simulink model "REGISTROS_64_BITS_01"  (R2022a)
settings: Solver=VariableStepAuto  StartTime=0.0  StopTime=10.0  RelTol=1e-3
undefined symbols (not defined in the file or in its folder): xc7z010iclg225
libraries: hdlBasic x6608, vmcUtilities x1
(part 1 of 23)
settings Model: Creator=sebas  LastModifiedBy=sebas

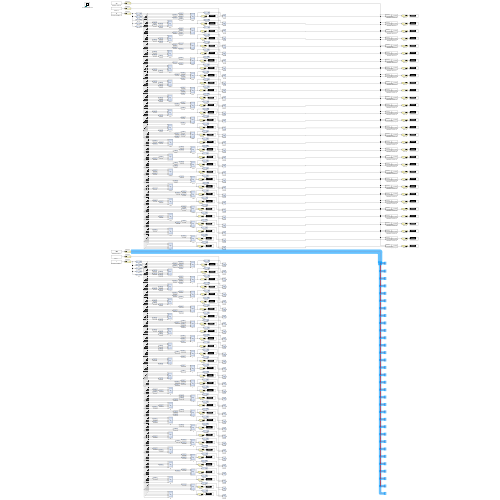
[thumbnail: Simulink's stored preview of the top-level diagram]
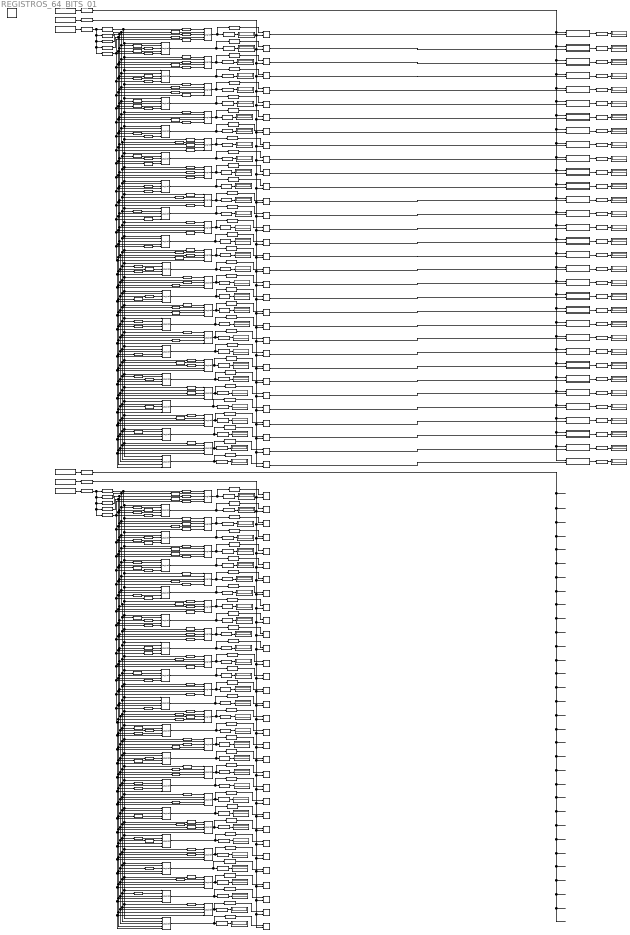
== system REGISTROS_64_BITS_01 ==
  00000 : hdlBasic/Logical  logical_function=AND  inputs=5  en=off  latency=0  precision=Full  arith_type=Unsigned  n_bits=16  bin_pt=0  align_bp=on  overflow=[]  quantization=[]  XmcBlockStatus=1  maskContainerNames=tabcontainer1  block_type=logical  block_config=sysgen:Logical_config
  00001 : hdlBasic/Logical  logical_function=AND  inputs=5  en=off  latency=0  precision=Full  arith_type=Unsigned  n_bits=16  bin_pt=0  align_bp=on  overflow=[]  quantization=[]  XmcBlockStatus=1  maskContainerNames=tabcontainer1  block_type=logical  block_config=sysgen:Logical_config
  00010 : hdlBasic/Logical  logical_function=AND  inputs=5  en=off  latency=0  precision=Full  arith_type=Unsigned  n_bits=16  bin_pt=0  align_bp=on  overflow=[]  quantization=[]  XmcBlockStatus=1  maskContainerNames=tabcontainer1  block_type=logical  block_config=sysgen:Logical_config
  00011 : hdlBasic/Logical  logical_function=AND  inputs=5  en=off  latency=0  precision=Full  arith_type=Unsigned  n_bits=16  bin_pt=0  align_bp=on  overflow=[]  quantization=[]  XmcBlockStatus=1  maskContainerNames=tabcontainer1  block_type=logical  block_config=sysgen:Logical_config
  00100 : hdlBasic/Logical  logical_function=AND  inputs=5  en=off  latency=0  precision=Full  arith_type=Unsigned  n_bits=16  bin_pt=0  align_bp=on  overflow=[]  quantization=[]  XmcBlockStatus=1  maskContainerNames=tabcontainer1  block_type=logical  block_config=sysgen:Logical_config
  00101 : hdlBasic/Logical  logical_function=AND  inputs=5  en=off  latency=0  precision=Full  arith_type=Unsigned  n_bits=16  bin_pt=0  align_bp=on  overflow=[]  quantization=[]  XmcBlockStatus=1  maskContainerNames=tabcontainer1  block_type=logical  block_config=sysgen:Logical_config
  00110 : hdlBasic/Logical  logical_function=AND  inputs=5  en=off  latency=0  precision=Full  arith_type=Unsigned  n_bits=16  bin_pt=0  align_bp=on  overflow=[]  quantization=[]  XmcBlockStatus=1  maskContainerNames=tabcontainer1  block_type=logical  block_config=sysgen:Logical_config
  00111 : hdlBasic/Logical  logical_function=AND  inputs=5  en=off  latency=0  precision=Full  arith_type=Unsigned  n_bits=16  bin_pt=0  align_bp=on  overflow=[]  quantization=[]  XmcBlockStatus=1  maskContainerNames=tabcontainer1  block_type=logical  block_config=sysgen:Logical_config
  01000 : hdlBasic/Logical  logical_function=AND  inputs=5  en=off  latency=0  precision=Full  arith_type=Unsigned  n_bits=16  bin_pt=0  align_bp=on  overflow=[]  quantization=[]  XmcBlockStatus=1  maskContainerNames=tabcontainer1  block_type=logical  block_config=sysgen:Logical_config
  01001 : hdlBasic/Logical  logical_function=AND  inputs=5  en=off  latency=0  precision=Full  arith_type=Unsigned  n_bits=16  bin_pt=0  align_bp=on  overflow=[]  quantization=[]  XmcBlockStatus=1  maskContainerNames=tabcontainer1  block_type=logical  block_config=sysgen:Logical_config
  01010 : hdlBasic/Logical  logical_function=AND  inputs=5  en=off  latency=0  precision=Full  arith_type=Unsigned  n_bits=16  bin_pt=0  align_bp=on  overflow=[]  quantization=[]  XmcBlockStatus=1  maskContainerNames=tabcontainer1  block_type=logical  block_config=sysgen:Logical_config
  01011 : hdlBasic/Logical  logical_function=AND  inputs=5  en=off  latency=0  precision=Full  arith_type=Unsigned  n_bits=16  bin_pt=0  align_bp=on  overflow=[]  quantization=[]  XmcBlockStatus=1  maskContainerNames=tabcontainer1  block_type=logical  block_config=sysgen:Logical_config
  01100 : hdlBasic/Logical  logical_function=AND  inputs=5  en=off  latency=0  precision=Full  arith_type=Unsigned  n_bits=16  bin_pt=0  align_bp=on  overflow=[]  quantization=[]  XmcBlockStatus=1  maskContainerNames=tabcontainer1  block_type=logical  block_config=sysgen:Logical_config
  01101 : hdlBasic/Logical  logical_function=AND  inputs=5  en=off  latency=0  precision=Full  arith_type=Unsigned  n_bits=16  bin_pt=0  align_bp=on  overflow=[]  quantization=[]  XmcBlockStatus=1  maskContainerNames=tabcontainer1  block_type=logical  block_config=sysgen:Logical_config
  01110 : hdlBasic/Logical  logical_function=AND  inputs=5  en=off  latency=0  precision=Full  arith_type=Unsigned  n_bits=16  bin_pt=0  align_bp=on  overflow=[]  quantization=[]  XmcBlockStatus=1  maskContainerNames=tabcontainer1  block_type=logical  block_config=sysgen:Logical_config
  01111 : hdlBasic/Logical  logical_function=AND  inputs=5  en=off  latency=0  precision=Full  arith_type=Unsigned  n_bits=16  bin_pt=0  align_bp=on  overflow=[]  quantization=[]  XmcBlockStatus=1  maskContainerNames=tabcontainer1  block_type=logical  block_config=sysgen:Logical_config
  {1..32,10000..10001,10010..10011,10100..10101,10110..10111,11000..11001,11010..11011,11100..11101,11110..11111} (48 alike) : hdlBasic/Logical  logical_function=AND  inputs=5  en=off  latency=0  precision=Full  arith_type=Unsigned  n_bits=16  bin_pt=0  align_bp=on  overflow=[]  quantization=[]  XmcBlockStatus=1  maskContainerNames=tabcontainer1  block_type=logical  block_config=sysgen:Logical_config
  BIT_00 : hdlBasic/Slice  nbits=1  boolean_output=off  mode=Lower Bit Location + Width  bit1=-3  base1=MSB of Input  bit0=0  base0=LSB of Input  XmcBlockStatus=1  maskContainerNames=group1  block_type=slice  block_config=sysgen:Slice_config
  BIT_01 : hdlBasic/Slice  nbits=1  boolean_output=off  mode=Lower Bit Location + Width  bit1=-2  base1=MSB of Input  bit0=1  base0=LSB of Input  XmcBlockStatus=1  maskContainerNames=group1  block_type=slice  block_config=sysgen:Slice_config
  BIT_02 : hdlBasic/Slice  nbits=1  boolean_output=off  mode=Lower Bit Location + Width  bit1=-3  base1=MSB of Input  bit0=2  base0=LSB of Input  XmcBlockStatus=1  maskContainerNames=group1  block_type=slice  block_config=sysgen:Slice_config
  BIT_03 : hdlBasic/Slice  nbits=1  boolean_output=off  mode=Lower Bit Location + Width  bit1=-2  base1=MSB of Input  bit0=3  base0=LSB of Input  XmcBlockStatus=1  maskContainerNames=group1  block_type=slice  block_config=sysgen:Slice_config
  BIT_04 : hdlBasic/Slice  nbits=1  boolean_output=off  mode=Lower Bit Location + Width  bit1=-2  base1=MSB of Input  bit0=4  base0=LSB of Input  XmcBlockStatus=1  maskContainerNames=group1  block_type=slice  block_config=sysgen:Slice_config
  BIT_1 : hdlBasic/Slice  nbits=1  boolean_output=off  mode=Lower Bit Location + Width  bit1=-3  base1=MSB of Input  bit0=0  base0=LSB of Input  XmcBlockStatus=1  maskContainerNames=group1  block_type=slice  block_config=sysgen:Slice_config
  BIT_2 : hdlBasic/Slice  nbits=1  boolean_output=off  mode=Lower Bit Location + Width  bit1=-2  base1=MSB of Input  bit0=1  base0=LSB of Input  XmcBlockStatus=1  maskContainerNames=group1  block_type=slice  block_config=sysgen:Slice_config
  BIT_3 : hdlBasic/Slice  nbits=1  boolean_output=off  mode=Lower Bit Location + Width  bit1=-3  base1=MSB of Input  bit0=2  base0=LSB of Input  XmcBlockStatus=1  maskContainerNames=group1  block_type=slice  block_config=sysgen:Slice_config
  BIT_4 : hdlBasic/Slice  nbits=1  boolean_output=off  mode=Lower Bit Location + Width  bit1=-2  base1=MSB of Input  bit0=3  base0=LSB of Input  XmcBlockStatus=1  maskContainerNames=group1  block_type=slice  block_config=sysgen:Slice_config
  BIT_5 : hdlBasic/Slice  nbits=1  boolean_output=off  mode=Lower Bit Location + Width  bit1=-2  base1=MSB of Input  bit0=4  base0=LSB of Input  XmcBlockStatus=1  maskContainerNames=group1  block_type=slice  block_config=sysgen:Slice_config
  Convert{,1..63} (64 alike) : hdlBasic/Convert  gui_display_data_type=Boolean  arith_type=Boolean  n_bits=16  bin_pt=14  float_type=Single  exp_bits=8  fraction_bits=24  quantization=Truncate  overflow=Wrap  en=off  latency=0  pipeline=off  XmcBlockStatus=1  maskContainerNames=group2  block_type=convert  block_config=sysgen:Convert_config  block_width=595  block_height=885
  Display{1..96} (96 alike) : Display
      Display38 settings: Format=decimal (Stored Integer)
      Display39 settings: Format=decimal (Stored Integer)
      Display40 settings: Format=decimal (Stored Integer)
      Display41 settings: Format=decimal (Stored Integer)
      Display42 settings: Format=decimal (Stored Integer)
      Display43 settings: Format=decimal (Stored Integer)
      Display44 settings: Format=decimal (Stored Integer)
      Display45 settings: Format=decimal (Stored Integer)
      Display46 settings: Format=decimal (Stored Integer)
      Display47 settings: Format=decimal (Stored Integer)
      Display48 settings: Format=decimal (Stored Integer)
      Display49 settings: Format=decimal (Stored Integer)
      Display50 settings: Format=decimal (Stored Integer)
      Display51 settings: Format=decimal (Stored Integer)
      Display52 settings: Format=decimal (Stored Integer)
      Display53 settings: Format=decimal (Stored Integer)
      Display54 settings: Format=decimal (Stored Integer)
      Display55 settings: Format=decimal (Stored Integer)
      Display56 settings: Format=decimal (Stored Integer)
      Display57 settings: Format=decimal (Stored Integer)
      Display58 settings: Format=decimal (Stored Integer)
      Display59 settings: Format=decimal (Stored Integer)
      Display60 settings: Format=decimal (Stored Integer)
      Display61 settings: Format=decimal (Stored Integer)
      Display62 settings: Format=decimal (Stored Integer)
      Display63 settings: Format=decimal (Stored Integer)
      Display64 settings: Format=decimal (Stored Integer)
      Display65 settings: Format=decimal (Stored Integer)
      Display66 settings: Format=decimal (Stored Integer)
      Display67 settings: Format=decimal (Stored Integer)
      Display68 settings: Format=decimal (Stored Integer)
      Display88 settings: Format=decimal (Stored Integer)
  Gateway In1 : hdlBasic/Gateway In  gui_display_data_type=Boolean  arith_type=Boolean  n_bits=1  bin_pt=0  preci_type=Single  exp_width=8  frac_width=24  rows=1  columns=1  quantization="Round  (unbiased: +/- Inf)"  overflow=Saturate  period=1  UseAsADC=off  ADCChannel='1'  interface=None  automatic_assignment=on  address_offset=hex2dec('00')  intf_name=''  intf_description=''  default_value=0  timing_constraint=None  locs_specified=off  LOCs={}  io_standard={}  inherit_from_input=off  hdl_port=on  XmcBlockStatus=1  maskContainerNames=group4  block_type=gatewayin  block_config=sysgen:gateway_in_config  block_width_w=590  block_height_w=620  block_width=640  block_height=850
  Gateway In2 : hdlBasic/Gateway In  gui_display_data_type=Fixed-point  arith_type=Signed (2's comp)  n_bits=64  bin_pt=0  preci_type=Single  exp_width=8  frac_width=24  rows=1  columns=1  quantization="Round  (unbiased: +/- Inf)"  overflow=Saturate  period=1  UseAsADC=off  ADCChannel='1'  interface=None  automatic_assignment=on  address_offset=hex2dec('00')  intf_name=''  intf_description=''  default_value=0  timing_constraint=None  locs_specified=off  LOCs={}  io_standard={}  inherit_from_input=off  hdl_port=on  XmcBlockStatus=1  maskContainerNames=group4  block_type=gatewayin  block_config=sysgen:gateway_in_config  block_width_w=590  block_height_w=620  block_width=640  block_height=850
  Gateway In3 : hdlBasic/Gateway In  gui_display_data_type=Boolean  arith_type=Boolean  n_bits=1  bin_pt=0  preci_type=Single  exp_width=8  frac_width=24  rows=1  columns=1  quantization="Round  (unbiased: +/- Inf)"  overflow=Saturate  period=1  UseAsADC=off  ADCChannel='1'  interface=None  automatic_assignment=on  address_offset=hex2dec('00')  intf_name=''  intf_description=''  default_value=0  timing_constraint=None  locs_specified=off  LOCs={}  io_standard={}  inherit_from_input=off  hdl_port=on  XmcBlockStatus=1  maskContainerNames=group4  block_type=gatewayin  block_config=sysgen:gateway_in_config  block_width_w=590  block_height_w=620  block_width=640  block_height=850
  Gateway In4 : hdlBasic/Gateway In  gui_display_data_type=Fixed-point  arith_type=Signed (2's comp)  n_bits=64  bin_pt=0  preci_type=Single  exp_width=8  frac_width=24  rows=1  columns=1  quantization="Round  (unbiased: +/- Inf)"  overflow=Saturate  period=1  UseAsADC=off  ADCChannel='1'  interface=None  automatic_assignment=on  address_offset=hex2dec('00')  intf_name=''  intf_description=''  default_value=0  timing_constraint=None  locs_specified=off  LOCs={}  io_standard={}  inherit_from_input=off  hdl_port=on  XmcBlockStatus=1  maskContainerNames=group4  block_type=gatewayin  block_config=sysgen:gateway_in_config  block_width_w=590  block_height_w=620  block_width=640  block_height=850
  Gateway In5 : hdlBasic/Gateway In  gui_display_data_type=Fixed-point  arith_type=Unsigned  n_bits=5  bin_pt=0  preci_type=Single  exp_width=8  frac_width=24  rows=1  columns=1  quantization="Round  (unbiased: +/- Inf)"  overflow=Saturate  period=1  UseAsADC=off  ADCChannel='1'  interface=None  automatic_assignment=on  address_offset=hex2dec('00')  intf_name=''  intf_description=''  default_value=0  timing_constraint=None  locs_specified=off  LOCs={}  io_standard={}  inherit_from_input=off  hdl_port=on  XmcBlockStatus=1  maskContainerNames=group4  block_type=gatewayin  block_config=sysgen:gateway_in_config  block_width_w=590  block_height_w=620  block_width=640  block_height=850
  Gateway In9 : hdlBasic/Gateway In  gui_display_data_type=Fixed-point  arith_type=Unsigned  n_bits=5  bin_pt=0  preci_type=Single  exp_width=8  frac_width=24  rows=1  columns=1  quantization="Round  (unbiased: +/- Inf)"  overflow=Saturate  period=1  UseAsADC=off  ADCChannel='1'  interface=None  automatic_assignment=on  address_offset=hex2dec('00')  intf_name=''  intf_description=''  default_value=0  timing_constraint=None  locs_specified=off  LOCs={}  io_standard={}  inherit_from_input=off  hdl_port=on  XmcBlockStatus=1  maskContainerNames=group4  block_type=gatewayin  block_config=sysgen:gateway_in_config  block_width_w=590  block_height_w=620  block_width=640  block_height=850
  Inverter{1..160} (160 alike) : hdlBasic/Inverter  en=off  latency=0  XmcBlockStatus=1  maskContainerNames=group2  block_type=inv  block_config=sysgen:Inverter_config
  Logical{,1..63} (64 alike) : hdlBasic/Logical  logical_function=AND  inputs=2  en=off  latency=0  precision=Full  arith_type=Unsigned  n_bits=16  bin_pt=0  align_bp=on  overflow=[]  quantization=[]  XmcBlockStatus=1  maskContainerNames=tabcontainer1  block_type=logical  block_config=sysgen:Logical_config
  REGISTER_DATA_00 : Constant  Value=99985
  REGISTER_DATA_1 : Constant  Value=99985
  REGISTER_NUMBER_00 : Constant  Value=30
  REGISTER_NUMBER_1 : Constant  Value=30
  REGISTRO_64_BITS_00 : Subsystem
  REGISTRO_64_BITS_1 : Subsystem
  REGISTRO_64_BITS_10 : Subsystem
  REGISTRO_64_BITS_11 : Subsystem
  REGISTRO_64_BITS_12 : Subsystem
  REGISTRO_64_BITS_13 : Subsystem
  REGISTRO_64_BITS_14 : Subsystem
  REGISTRO_64_BITS_15 : Subsystem
  REGISTRO_64_BITS_16 : Subsystem
  REGISTRO_64_BITS_17 : Subsystem
  REGISTRO_64_BITS_18 : Subsystem
  REGISTRO_64_BITS_19 : Subsystem
  REGISTRO_64_BITS_2 : Subsystem
  REGISTRO_64_BITS_20 : Subsystem
  REGISTRO_64_BITS_21 : Subsystem
  REGISTRO_64_BITS_22 : Subsystem
  REGISTRO_64_BITS_23 : Subsystem
  REGISTRO_64_BITS_24 : Subsystem
  REGISTRO_64_BITS_25 : Subsystem
  REGISTRO_64_BITS_26 : Subsystem
  REGISTRO_64_BITS_27 : Subsystem
  REGISTRO_64_BITS_28 : Subsystem
  REGISTRO_64_BITS_29 : Subsystem
  REGISTRO_64_BITS_3 : Subsystem
  REGISTRO_64_BITS_30 : Subsystem
  REGISTRO_64_BITS_31 : Subsystem
  REGISTRO_64_BITS_4 : Subsystem
  REGISTRO_64_BITS_5 : Subsystem
  REGISTRO_64_BITS_6 : Subsystem
  REGISTRO_64_BITS_7 : Subsystem
  REGISTRO_64_BITS_8 : Subsystem
  REGISTRO_64_BITS_9 : Subsystem
  Result{1..64} (64 alike) : hdlBasic/Gateway Out  inherit_from_input=off  hdl_port=on  rows=1  columns=1  UseAsDAC=off  DACChannel='1'  interface=None  automatic_assignment=on  address_offset=hex2dec('00')  intf_name=''  intf_description=''  timing_constraint=None  locs_specified=off  LOCs={}  io_standard={}  XmcBlockStatus=1  maskContainerNames=group4  block_type=gatewayout  block_config=sysgen:gateway_out_config  block_width_w=590  block_height_w=620  block_width=620  block_height=750
  Result_{1..32} (32 alike) : hdlBasic/Gateway Out  inherit_from_input=off  hdl_port=on  rows=1  columns=1  UseAsDAC=off  DACChannel='1'  interface=None  automatic_assignment=on  address_offset=hex2dec('00')  intf_name=''  intf_description=''  timing_constraint=None  locs_specified=off  LOCs={}  io_standard={}  XmcBlockStatus=1  maskContainerNames=group4  block_type=gatewayout  block_config=sysgen:gateway_out_config  block_width_w=590  block_height_w=620  block_width=620  block_height=750
  Vitis Model Composer Hub : vmcUtilities/Vitis Model Composer Hub  Tag=genX  CodeGeneration=off  TargetDirectory=./code  ExportType=AI Engines  IpVendor=xilinx.com  IpLibrary=hls  IpVersion=1.0  IpHWLanguage=Verilog  AieCompilerOptions={}  AieSimulatorOptions={}  CreateTestbench=off  TestbenchStackSize=10  RunAieSim=off  AieSimTimeout=50000  RunAieSimProfiling=off  LaunchVitisAnalyzer=off  PlotOutput=off  RunX86Sim=off  X86SimTimeout=10  GenHwImage=off  PlatformType=Not Specified  HwSystemType=Baremetal  HwValidationTarget=hw  ProjDevice=xc7z010iclg225-1L  ProjDevicePart=xc7z010iclg225-1L  SamplePeriod=-1  ClockFrequency=200  DataPathParallelism=1  xilinxfamily=zynq  part=xc7z010i  speed=-1L  package=clg225  directory=./netlist  testbench=off  incr_netlist=off  synthesis_tool=Vivado  clock_wrapper=Clock Enables  dbl_ovrd=According to Block Masks  dcm_input_clock_period=10  sysclk_period=10  simulink_period=1  eval_field=0  LogFileName=''  NThreads=4
  WRITE_00 : Constant
  WRITE_1 : Constant
  wires:
  11000/1 -> Convert7/1, Result30/1
  01001/1 -> Convert22/1, Result19/1
  Inverter34/1 -> 00111/4
  Inverter43/1 -> 01011/3
  Inverter26/1 -> 01001/2
  Inverter75/1 -> 11010/3
  Inverter59/1 -> 01110/5
  Inverter38/1 -> 01000/2
  Result36/1 -> Display36/1
  Result27/1 -> Display27/1
  00111/1 -> Convert24/1, Result13/1
  Inverter12/1 -> 00011/3
  Inverter61/1 -> 10101/2
  Inverter6/1 -> 00001/5
  Result15/1 -> Display15/1
  01011/1 -> Convert20/1, Result21/1
  Result18/1 -> Display18/1
  Result20/1 -> Display20/1
  Result17/1 -> Display17/1
  Inverter47/1 -> 11001/3
  Result6/1 -> Display6/1
  Inverter71/1 -> 10000/4
  Inverter9/1 -> 00001/4
  Inverter84/1 -> 11011/3
  Result8/1 -> Display8/1
  BIT_00/1 -> 01001/1, 01011/1, 01101/1, 01111/1, 11001/1, 11011/1, 11101/1, 11111/1, Inverter94/1, Inverter89/1, Inverter83/1, Inverter82/1, 10111/1, Inverter73/1, 10101/1, Inverter58/1, 10011/1, Inverter45/1, 10001/1, Inverter72/1, Inverter62/1, Inverter52/1, Inverter42/1, Inverter40/1, 00111/1, Inverter30/1, 00101/1, Inverter21/1, 00011/1, Inverter14/1, 00001/1, Inverter8/1
  Inverter17/1 -> 00011/4
  Inverter78/1 -> 11000/3
  01111/1 -> Convert16/1, Result17/1
  Inverter5/1 -> 00001/3
  Inverter80/1 -> 11000/2
  Inverter32/1 -> 00111/5
  Inverter24/1 -> 00101/4
  00011/1 -> Convert28/1, Result9/1
  11101/1 -> Convert2/1, Result27/1
  00001/1 -> Convert30/1, Result7/1
  Inverter83/1 -> 11010/1
  Inverter28/1 -> 10010/3
  01110/1 -> Convert17/1, Result16/1
  Inverter23/1 -> 00101/2
  Logical2/1 -> REGISTRO_64_BITS_2/2(C - ENABLE (1 BIT))
  Result10/1 -> Display10/1
  Logical7/1 -> REGISTRO_64_BITS_7/2(C - ENABLE (1 BIT))
  Inverter72/1 -> 10000/1
  Convert17/1 -> Logical14/1
  Inverter91/1 -> 11101/2
  Logical20/1 -> REGISTRO_64_BITS_28/2(C - ENABLE (1 BIT))
  Result_23/1 -> Display57/1
  Logical23/1 -> REGISTRO_64_BITS_31/2(C - ENABLE (1 BIT))
  Result22/1 -> Display22/1
  REGISTRO_64_BITS_22/1(Q (64 BIT)) -> Result_24/1
  Result14/1 -> Display14/1
  Result12/1 -> Display12/1
  REGISTRO_64_BITS_19/1(Q (64 BIT)) -> Result_19/1
  Result29/1 -> Display29/1
  Logical10/1 -> REGISTRO_64_BITS_10/2(C - ENABLE (1 BIT))
  Result32/1 -> Display32/1
  11011/1 -> Convert4/1, Result33/1
  Result30/1 -> Display30/1
  REGISTER_NUMBER_00/1 -> Gateway In9/1
  Inverter7/1 -> 00001/2
  Logical6/1 -> REGISTRO_64_BITS_6/2(C - ENABLE (1 BIT))
  Result_18/1 -> Display60/1
  REGISTRO_64_BITS_5/1(Q (64 BIT)) -> Result_5/1
  Inverter3/1 -> 00000/2
  Logical12/1 -> REGISTRO_64_BITS_12/2(C - ENABLE (1 BIT))
  Logical19/1 -> REGISTRO_64_BITS_27/2(C - ENABLE (1 BIT))
  Result19/1 -> Display19/1
  REGISTRO_64_BITS_29/1(Q (64 BIT)) -> Result_29/1
  Logical13/1 -> REGISTRO_64_BITS_13/2(C - ENABLE (1 BIT))
  Inverter49/1 -> 01100/5
  Logical11/1 -> REGISTRO_64_BITS_11/2(C - ENABLE (1 BIT))
  Result_12/1 -> Display47/1
  Logical9/1 -> REGISTRO_64_BITS_9/2(C - ENABLE (1 BIT))
  Result25/1 -> Display25/1
  Convert22/1 -> Logical9/1
  Result33/1 -> Display33/1
  Inverter8/1 -> 00000/1
  Logical17/1 -> REGISTRO_64_BITS_17/2(C - ENABLE (1 BIT))
  Result_21/1 -> Display56/1
  Logical30/1 -> REGISTRO_64_BITS_24/2(C - ENABLE (1 BIT))
  REGISTRO_64_BITS_16/1(Q (64 BIT)) -> Result_18/1
  Logical18/1 -> REGISTRO_64_BITS_26/2(C - ENABLE (1 BIT))
  Inverter52/1 -> 01100/1
  REGISTRO_64_BITS_30/1(Q (64 BIT)) -> Result_32/1
  Logical26/1 -> REGISTRO_64_BITS_20/2(C - ENABLE (1 BIT))
  01000/1 -> Convert23/1, Result18/1
  Logical25/1 -> REGISTRO_64_BITS_19/2(C - ENABLE (1 BIT))
  REGISTRO_64_BITS_3/1(Q (64 BIT)) -> Result_3/1
  Inverter42/1 -> 01010/1
  Inverter68/1 -> 10000/3
  Logical21/1 -> REGISTRO_64_BITS_29/2(C - ENABLE (1 BIT))
  Inverter66/1 -> 11001/2
  Inverter73/1 -> 10110/1
  Inverter11/1 -> 00010/5
  Result_29/1 -> Display64/1
  Convert6/1 -> Logical31/1
  Inverter35/1 -> 01010/5
  REGISTRO_64_BITS_31/1(Q (64 BIT)) -> Result_31/1
  Convert5/1 -> Logical18/1
  Inverter4/1 -> 00000/4
  REGISTRO_64_BITS_20/1(Q (64 BIT)) -> Result_22/1
  REGISTRO_64_BITS_8/1(Q (64 BIT)) -> Result_10/1
  REGISTRO_64_BITS_1/1(Q (64 BIT)) -> Result_1/1
  Convert28/1 -> Logical3/1
  REGISTRO_64_BITS_21/1(Q (64 BIT)) -> Result_21/1
  Convert25/1 -> Logical6/1
  REGISTRO_64_BITS_12/1(Q (64 BIT)) -> Result_14/1
  REGISTRO_64_BITS_26/1(Q (64 BIT)) -> Result_28/1
  Inverter19/1 -> 00100/2
  Result_11/1 -> Display46/1
  Logical31/1 -> REGISTRO_64_BITS_25/2(C - ENABLE (1 BIT))
  REGISTRO_64_BITS_11/1(Q (64 BIT)) -> Result_11/1
  Result_28/1 -> Display63/1
  REGISTRO_64_BITS_7/1(Q (64 BIT)) -> Result_7/1
  Result31/1 -> Display31/1
  Gateway In2/1 -> REGISTRO_64_BITS_00/1(D (64 BIT)), REGISTRO_64_BITS_1/1(D (64 BIT)), REGISTRO_64_BITS_2/1(D (64 BIT)), REGISTRO_64_BITS_3/1(D (64 BIT)), REGISTRO_64_BITS_4/1(D (64 BIT)), REGISTRO_64_BITS_5/1(D (64 BIT)), REGISTRO_64_BITS_6/1(D (64 BIT)), REGISTRO_64_BITS_7/1(D (64 BIT)), REGISTRO_64_BITS_8/1(D (64 BIT)), REGISTRO_64_BITS_9/1(D (64 BIT)), REGISTRO_64_BITS_10/1(D (64 BIT)), REGISTRO_64_BITS_11/1(D (64 BIT)), REGISTRO_64_BITS_12/1(D (64 BIT)), REGISTRO_64_BITS_13/1(D (64 BIT)), REGISTRO_64_BITS_14/1(D (64 BIT)), REGISTRO_64_BITS_15/1(D (64 BIT)), REGISTRO_64_BITS_16/1(D (64 BIT)), REGISTRO_64_BITS_17/1(D (64 BIT)), REGISTRO_64_BITS_18/1(D (64 BIT)), REGISTRO_64_BITS_19/1(D (64 BIT)), REGISTRO_64_BITS_20/1(D (64 BIT)), REGISTRO_64_BITS_21/1(D (64 BIT)), REGISTRO_64_BITS_22/1(D (64 BIT)), REGISTRO_64_BITS_23/1(D (64 BIT)), REGISTRO_64_BITS_24/1(D (64 BIT)), REGISTRO_64_BITS_25/1(D (64 BIT)), REGISTRO_64_BITS_26/1(D (64 BIT)), REGISTRO_64_BITS_27/1(D (64 BIT)), REGISTRO_64_BITS_28/1(D (64 BIT)), REGISTRO_64_BITS_29/1(D (64 BIT)), REGISTRO_64_BITS_31/1(D (64 BIT)), REGISTRO_64_BITS_30/1(D (64 BIT))
  REGISTRO_64_BITS_13/1(Q (64 BIT)) -> Result_13/1
  Result21/1 -> Display21/1
  Result_25/1 -> Display61/1
  Convert20/1 -> Logical11/1
  Inverter16/1 -> 01001/3
  Result_16/1 -> Display50/1
  REGISTRO_64_BITS_27/1(Q (64 BIT)) -> Result_27/1
  Result_19/1 -> Display54/1
  Convert26/1 -> Logical5/1
  Convert3/1 -> Logical20/1
  Inverter101/1 -> 10001/4
  Convert31/1 -> Logical/1
  Convert23/1 -> Logical8/1
  Inverter87/1 -> 10001/3
  Convert12/1 -> Logical25/1
  Inverter64/1 -> 01111/5
  Convert24/1 -> Logical7/1
  Convert19/1 -> Logical12/1
  Convert14/1 -> Logical17/1
  Convert16/1 -> Logical15/1
  REGISTRO_64_BITS_28/1(Q (64 BIT)) -> Result_30/1
  Convert10/1 -> Logical27/1
  Result7/1 -> Display7/1
  Result35/1 -> Display35/1
  Result_6/1 -> Display44/1
  Inverter36/1 -> 01000/3
  Inverter22/1 -> 00101/5
  Result_27/1 -> Display62/1
  Convert9/1 -> Logical28/1
  Result_10/1 -> Display52/1
  Result_9/1 -> Display45/1
  Result_20/1 -> Display55/1
  Result_13/1 -> Display48/1
  Result_22/1 -> Display59/1
  Result_24/1 -> Display58/1
  Result9/1 -> Display9/1
  Convert27/1 -> Logical4/1
  01100/1 -> Convert19/1, Result14/1
  Result_4/1 -> Display40/1
  Result_14/1 -> Display51/1
  REGISTRO_64_BITS_14/1(Q (64 BIT)) -> Result_16/1
  Inverter88/1 -> 11100/2
  Gateway In9/1 -> BIT_02/1, BIT_03/1, BIT_04/1, BIT_01/1, BIT_00/1
  00000/1 -> Convert31/1, Result6/1
  Inverter45/1 -> 10010/1
  Result_30/1 -> Display67/1
  REGISTRO_64_BITS_00/1(Q (64 BIT)) -> Result_2/1
  Result_17/1 -> Display53/1
  10010/1 -> Convert13/1, Result36/1
  10100/1 -> Convert11/1, Result22/1
  10110/1 -> Convert9/1, Result24/1
  Inverter62/1 -> 01110/1
  10000/1 -> Convert15/1, Result34/1
  01101/1 -> Convert18/1, Result15/1
  Result23/1 -> Display23/1
  Logical27/1 -> REGISTRO_64_BITS_21/2(C - ENABLE (1 BIT))
  Convert21/1 -> Logical10/1
  Inverter40/1 -> 01000/1
  00110/1 -> Convert25/1, Result12/1
  11010/1 -> Convert5/1, Result32/1
  BIT_03/1 -> Inverter20/1, Inverter24/1, Inverter29/1, Inverter34/1, 01100/4, 01101/4, 01110/4, 01111/4, Inverter57/1, Inverter63/1, Inverter69/1, Inverter76/1, 11100/4, 11101/4, 11110/4, 11111/4, 11011/4, 11010/4, 11001/4, 11000/4, Inverter48/1, Inverter41/1, Inverter101/1, Inverter71/1, 01011/4, 01010/4, 01001/4, 01000/4, Inverter17/1, Inverter13/1, Inverter9/1, Inverter4/1
  Result_15/1 -> Display49/1
  Result37/1 -> Display37/1
  Inverter13/1 -> 00010/4
  Result_5/1 -> Display41/1
  REGISTRO_64_BITS_6/1(Q (64 BIT)) -> Result_8/1
  Logical5/1 -> REGISTRO_64_BITS_5/2(C - ENABLE (1 BIT))
  Inverter58/1 -> 10100/1
  11001/1 -> Convert6/1, Result31/1
  REGISTRO_64_BITS_24/1(Q (64 BIT)) -> Result_26/1
  REGISTRO_64_BITS_25/1(Q (64 BIT)) -> Result_25/1
  Result_8/1 -> Display43/1
  Inverter21/1 -> 00100/1
  Inverter48/1 -> 10011/4
  Inverter14/1 -> 00010/1
  Inverter50/1 -> 01100/2
  Logical22/1 -> REGISTRO_64_BITS_30/2(C - ENABLE (1 BIT))
  Logical1/1 -> REGISTRO_64_BITS_1/2(C - ENABLE (1 BIT))
  Inverter53/1 -> 10100/2
  Inverter20/1 -> 00100/4
  BIT_04/1 -> Inverter15/1, Inverter18/1, Inverter25/1, Inverter35/1, Inverter44/1, Inverter49/1, Inverter54/1, Inverter59/1, Inverter64/1, 10100/5, 10110/5, 11000/5, 11001/5, 11010/5, 11011/5, 11100/5, 11101/5, 11110/5, 11111/5, 10111/5, 10101/5, 10011/5, 10010/5, 10001/5, 10000/5, Inverter37/1, Inverter32/1, Inverter27/1, Inverter22/1, Inverter11/1, Inverter2/1, Inverter6/1
  BIT_01/1 -> 00010/2, 00011/2, Inverter19/1, Inverter23/1, 00111/2, Inverter26/1, 01011/2, Inverter50/1, Inverter55/1, 01111/2, 10010/2, 10011/2, Inverter53/1, Inverter61/1, 10111/2, Inverter66/1, 11011/2, Inverter88/1, Inverter91/1, 11111/2, 11110/2, 11010/2, Inverter80/1, 10110/2, Inverter97/1, Inverter70/1, 01110/2, 01010/2, Inverter38/1, 00110/2, Inverter7/1, Inverter3/1
  Convert1/1 -> Logical22/1
  Inverter39/1 -> 10011/3
  Logical15/1 -> REGISTRO_64_BITS_15/2(C - ENABLE (1 BIT))
  Convert29/1 -> Logical2/1
  BIT_02/1 -> Inverter10/1, Inverter12/1, 01110/3, 01111/3, Inverter28/1, Inverter39/1, 11110/3, 11111/3, 11101/3, 11100/3, Inverter84/1, Inverter75/1, Inverter47/1, Inverter78/1, 10111/3, 10110/3, 10101/3, 10100/3, Inverter87/1, Inverter68/1, 01101/3, 01100/3, Inverter43/1, Inverter33/1, Inverter16/1, Inverter36/1, 00111/3, 00110/3, 00101/3, 00100/3, Inverter5/1, Inverter1/1
  Inverter37/1 -> 01000/5
  Inverter41/1 -> 10010/4
  Inverter27/1 -> 00110/5
  Convert8/1 -> Logical29/1
  Inverter2/1 -> 00000/5
  Convert18/1 -> Logical13/1
  Inverter1/1 -> 00000/3
  00101/1 -> Convert26/1, Result11/1
  Logical14/1 -> REGISTRO_64_BITS_14/2(C - ENABLE (1 BIT))
  00010/1 -> Convert29/1, Result8/1
  10001/1 -> Convert14/1, Result35/1
  Logical28/1 -> REGISTRO_64_BITS_22/2(C - ENABLE (1 BIT))
  REGISTRO_64_BITS_4/1(Q (64 BIT)) -> Result_6/1
  Result_7/1 -> Display42/1
  Inverter63/1 -> 10101/4
  REGISTRO_64_BITS_17/1(Q (64 BIT)) -> Result_17/1
  Inverter82/1 -> 11000/1
  Inverter89/1 -> 11100/1
  Inverter70/1 -> 10000/2
  Logical24/1 -> REGISTRO_64_BITS_18/2(C - ENABLE (1 BIT))
  Result16/1 -> Display16/1
  Convert/1 -> Logical23/1
  Result_3/1 -> Display39/1
  Inverter76/1 -> 10111/4
  Convert7/1 -> Logical30/1
  Inverter30/1 -> 00110/1
  Result34/1 -> Display34/1
  Result_32/1 -> Display66/1
  Result26/1 -> Display26/1
  REGISTRO_64_BITS_9/1(Q (64 BIT)) -> Result_9/1
  Result13/1 -> Display13/1
  00100/1 -> Convert27/1, Result10/1
  Result24/1 -> Display24/1
  Convert15/1 -> Logical16/1
  Inverter55/1 -> 01101/2
  Logical16/1 -> REGISTRO_64_BITS_16/2(C - ENABLE (1 BIT))
  Result_26/1 -> Display68/1
  Logical3/1 -> REGISTRO_64_BITS_3/2(C - ENABLE (1 BIT))
  Inverter57/1 -> 10100/4
  REGISTRO_64_BITS_23/1(Q (64 BIT)) -> Result_23/1
  Inverter54/1 -> 01101/5
  REGISTRO_64_BITS_15/1(Q (64 BIT)) -> Result_15/1
  Logical8/1 -> REGISTRO_64_BITS_8/2(C - ENABLE (1 BIT))
  Logical29/1 -> REGISTRO_64_BITS_23/2(C - ENABLE (1 BIT))
  Inverter29/1 -> 00110/4
  Inverter25/1 -> 01001/5
  REGISTER_DATA_00/1 -> Gateway In2/1
  Result_2/1 -> Display88/1
  11110/1 -> Convert1/1, Result28/1
  Inverter18/1 -> 00100/5
  Convert4/1 -> Logical19/1
  REGISTRO_64_BITS_2/1(Q (64 BIT)) -> Result_4/1
  Inverter33/1 -> 01010/3
  Result_31/1 -> Display65/1
  10111/1 -> Convert8/1, Result25/1
  Logical/1 -> REGISTRO_64_BITS_00/2(C - ENABLE (1 BIT))
  Inverter69/1 -> 10110/4
  REGISTRO_64_BITS_18/1(Q (64 BIT)) -> Result_20/1
  Convert30/1 -> Logical1/1
  Inverter44/1 -> 01011/5
  Gateway In1/1 -> Logical13/2, Logical15/2, Logical30/2, Logical20/2, Logical21/2, Logical23/2, Logical22/2, Logical19/2, Logical18/2, Logical31/2, Logical29/2, Logical28/2, Logical27/2, Logical26/2, Logical25/2, Logical24/2, Logical17/2, Logical16/2, Logical14/2, Logical12/2, Logical11/2, Logical10/2, Logical9/2, Logical8/2, Logical7/2, Logical6/2, Logical5/2, Logical4/2, Logical3/2, Logical2/2, Logical1/2, Logical/2
  Inverter97/1 -> 10001/2
  Inverter94/1 -> 11110/1
  REGISTRO_64_BITS_10/1(Q (64 BIT)) -> Result_12/1
  Result28/1 -> Display28/1
  10011/1 -> Convert12/1, Result37/1
  Result_1/1 -> Display38/1
  Inverter15/1 -> 00011/5
  11111/1 -> Convert/1, Result29/1
  Result11/1 -> Display11/1
  11100/1 -> Convert3/1, Result26/1
  01010/1 -> Convert21/1, Result20/1
  10101/1 -> Convert10/1, Result23/1
  Convert2/1 -> Logical21/1
  Logical4/1 -> REGISTRO_64_BITS_4/2(C - ENABLE (1 BIT))
  Inverter10/1 -> 00010/3
  Convert11/1 -> Logical26/1
  WRITE_00/1 -> Gateway In1/1
  Convert13/1 -> Logical24/1
  WRITE_1/1 -> Gateway In3/1
  Convert37/1 -> Logical49/1
  Inverter46/1 -> 3/3
  Result2/1 -> Display2/1
  Inverter74/1 -> 4/5
  32/1 -> Convert32/1, Result52/1
  Convert44/1 -> Logical46/1
  Inverter160/1 -> 18/2
  20/1 -> Convert36/1, Result60/1
  Convert56/1 -> Logical33/1
  Inverter119/1 -> 12/5
  Inverter107/1 -> 11/3
  Convert58/1 -> Logical43/1
  Inverter103/1 -> 7/4
  Inverter98/1 -> 10/5
  Inverter81/1 -> 5/5
  Inverter128/1 -> 14/5
  Result47/1 -> Display78/1
  Inverter130/1 -> 21/4
  Convert39/1 -> Logical40/1
  BIT_1/1 -> 10/1, 12/1, 14/1, 16/1, 26/1, 28/1, 30/1, 32/1, Inverter159/1, Inverter156/1, Inverter152/1, Inverter151/1, 24/1, Inverter145/1, 22/1, Inverter131/1, 20/1, Inverter120/1, 18/1, Inverter144/1, Inverter135/1, Inverter126/1, Inverter117/1, Inverter115/1, 8/1, Inverter105/1, 6/1, Inverter92/1, 4/1, Inverter67/1, 2/1, Inverter149/1
  Result49/1 -> Display80/1
  Convert61/1 -> Logical56/1
  Inverter147/1 -> 24/4
  Convert32/1 -> Logical48/1
  Convert35/1 -> Logical51/1
  Inverter142/1 -> 17/2
  Inverter151/1 -> 25/1
  18/1 -> Convert38/1, Result58/1
  Inverter136/1 -> 22/4
  Inverter116/1 -> 19/4
  Convert62/1 -> Logical54/1
  Inverter111/1 -> 9/5
  Convert42/1 -> Logical37/1
  Inverter129/1 -> 14/2
  Convert33/1 -> Logical47/1
  Convert54/1 -> Logical44/1
  Inverter113/1 -> 20/3
  24/1 -> Convert62/1, Result48/1
  Inverter140/1 -> 23/4
  Inverter90/1 -> 5/4
  26/1 -> Convert60/1, Result54/1
  Inverter92/1 -> 5/1
  Inverter127/1 -> 21/2
  Inverter67/1 -> 3/1
  Inverter131/1 -> 21/1
  22/1 -> Convert34/1, Result46/1
  21/1 -> Convert35/1, Result45/1
  Inverter105/1 -> 7/1
  Inverter135/1 -> 15/1
  11/1 -> Convert46/1, Result43/1
  29/1 -> Convert55/1, Result49/1
  Gateway In5/1 -> BIT_3/1, BIT_4/1, BIT_5/1, BIT_2/1, BIT_1/1
  Inverter120/1 -> 19/1
  1/1 -> Convert57/1, Result61/1
  Convert52/1 -> Logical58/1
  13/1 -> Convert43/1, Result5/1
  Convert63/1 -> Logical53/1
  Result58/1 -> Display90/1
  Convert34/1 -> Logical52/1
  Inverter110/1 -> 9/3
  Result62/1 -> Display94/1
  Inverter154/1 -> 18/3
  Gateway In3/1 -> Logical37/2, Logical39/2, Logical56/2, Logical45/2, Logical46/2, Logical48/2, Logical47/2, Logical43/2, Logical42/2, Logical57/2, Logical54/2, Logical53/2, Logical52/2, Logical51/2, Logical50/2, Logical49/2, Logical41/2, Logical40/2, Logical38/2, Logical36/2, Logical35/2, Logical34/2, Logical63/2, Logical62/2, Logical61/2, Logical60/2, Logical59/2, Logical58/2, Logical55/2, Logical44/2, Logical33/2, Logical32/2
  Inverter51/1 -> 18/4
  Convert36/1 -> Logical50/1
  Convert40/1 -> Logical39/1
  Convert49/1 -> Logical61/1
  Convert57/1 -> Logical32/1
  6/1 -> Convert51/1, Result2/1
  Convert48/1 -> Logical62/1
  Convert38/1 -> Logical41/1
  Convert43/1 -> Logical36/1
  Convert55/1 -> Logical45/1
  Inverter77/1 -> 10/3
  Gateway In4/1 -> ?
  Convert45/1 -> Logical35/1
  BIT_2/1 -> 3/2, 4/2, Inverter85/1, Inverter95/1, 8/2, Inverter99/1, 12/2, Inverter125/1, Inverter129/1, 16/2, 19/2, 20/2, Inverter127/1, Inverter134/1, 24/2, Inverter138/1, 28/2, Inverter155/1, Inverter158/1, 32/2, 31/2, 27/2, Inverter150/1, 23/2, Inverter160/1, Inverter142/1, 15/2, 11/2, Inverter112/1, 7/2, Inverter141/1, Inverter104/1
  REGISTER_DATA_1/1 -> Gateway In4/1
  31/1 -> Convert33/1, Result51/1
  7/1 -> Convert50/1, Result3/1
  Result60/1 -> Display92/1
  Inverter93/1 -> 6/5
  Inverter114/1 -> 1/4
  Convert59/1 -> Logical42/1
  Inverter109/1 -> 11/5
  Inverter145/1 -> 23/1
  27/1 -> Convert59/1, Result55/1
  Inverter31/1 -> 1/3
  Inverter117/1 -> 11/1
  Inverter139/1 -> 17/3
  Inverter56/1 -> 3/5
  Inverter149/1 -> 1/1
  Inverter156/1 -> 29/1
  9/1 -> Convert48/1, Result41/1
  Result56/1 -> Display87/1
  Inverter65/1 -> 3/4
  Inverter126/1 -> 13/1
  Result4/1 -> Display4/1
  Inverter104/1 -> 1/2
  Result48/1 -> Display79/1
  Result42/1 -> Display73/1
  Result52/1 -> Display83/1
  Result3/1 -> Display3/1
  Result55/1 -> Display86/1
  Inverter141/1 -> 2/2
  17/1 -> Convert39/1, Result57/1
  28/1 -> Convert58/1, Result56/1
  Inverter125/1 -> 13/2
  REGISTER_NUMBER_1/1 -> Gateway In5/1
  Convert41/1 -> Logical38/1
  Result1/1 -> Display1/1
  Inverter95/1 -> 6/2
  Result5/1 -> Display5/1
  Result45/1 -> Display76/1
  Inverter144/1 -> 17/1
  Result46/1 -> Display77/1
  Inverter158/1 -> 30/2
  4/1 -> Convert53/1, Result64/1
  Result64/1 -> Display96/1
  15/1 -> Convert41/1, Result39/1
  Inverter123/1 -> 13/5
  30/1 -> Convert44/1, Result50/1
  Inverter102/1 -> 19/3
  Inverter86/1 -> 1/5
  BIT_3/1 -> Inverter46/1, Inverter60/1, 15/3, 16/3, Inverter102/1, Inverter113/1, 31/3, 32/3, 30/3, 29/3, Inverter153/1, Inverter146/1, Inverter121/1, Inverter148/1, 24/3, 23/3, 22/3, 21/3, Inverter154/1, Inverter139/1, 14/3, 13/3, Inverter118/1, Inverter107/1, Inverter77/1, Inverter110/1, 8/3, 7/3, 6/3, 5/3, Inverter124/1, Inverter31/1
  Inverter100/1 -> 7/5
  Inverter96/1 -> 6/4
  16/1 -> Convert40/1, Result40/1
  Inverter106/1 -> 8/5
  Inverter124/1 -> 2/3
  Inverter79/1 -> 4/4
  Inverter150/1 -> 25/2
  Inverter157/1 -> 2/4
  Result61/1 -> Display93/1
  Convert46/1 -> Logical34/1
  Inverter148/1 -> 25/3
  Inverter143/1 -> 17/4
  Result63/1 -> Display95/1
  Inverter60/1 -> 4/3
  Inverter152/1 -> 27/1
  Inverter134/1 -> 22/2
  23/1 -> Convert63/1, Result47/1
  Result53/1 -> Display84/1
  Inverter122/1 -> 20/4
  12/1 -> Convert45/1, Result44/1
  Inverter121/1 -> 26/3
  Inverter138/1 -> 26/2
  Result40/1 -> Display71/1
  Inverter115/1 -> 9/1
  Result38/1 -> Display69/1
  Inverter132/1 -> 15/5
  25/1 -> Convert61/1, Result53/1
  Inverter118/1 -> 12/3
  Inverter99/1 -> 10/2
  10/1 -> Convert47/1, Result42/1
  Inverter108/1 -> 8/4
  Result44/1 -> Display75/1
  Convert53/1 -> Logical55/1
  Result50/1 -> Display81/1
  BIT_4/1 -> Inverter90/1, Inverter96/1, Inverter103/1, Inverter108/1, 13/4, 14/4, 15/4, 16/4, Inverter130/1, Inverter136/1, Inverter140/1, Inverter147/1, 29/4, 30/4, 31/4, 32/4, 28/4, 27/4, 26/4, 25/4, Inverter122/1, Inverter116/1, Inverter51/1, Inverter143/1, 12/4, 11/4, 10/4, 9/4, Inverter79/1, Inverter65/1, Inverter157/1, Inverter114/1
  Inverter153/1 -> 28/3
  Inverter85/1 -> 5/2
  Convert50/1 -> Logical60/1
  19/1 -> Convert37/1, Result59/1
  5/1 -> Convert52/1, Result1/1
  Convert47/1 -> Logical63/1
  Result59/1 -> Display91/1
  Result57/1 -> Display89/1
  Inverter159/1 -> 31/1
  Convert51/1 -> Logical59/1
  Result54/1 -> Display85/1
  2/1 -> Convert56/1, Result62/1
  8/1 -> Convert49/1, Result4/1
  Inverter146/1 -> 27/3
  Inverter137/1 -> 16/5
  3/1 -> Convert54/1, Result63/1
  Inverter155/1 -> 29/2
  Convert60/1 -> Logical57/1
  Result51/1 -> Display82/1
  Inverter133/1 -> 2/5
  Result43/1 -> Display74/1
  BIT_5/1 -> Inverter74/1, Inverter81/1, Inverter98/1, Inverter109/1, Inverter119/1, Inverter123/1, Inverter128/1, Inverter132/1, Inverter137/1, 21/5, 23/5, 25/5, 26/5, 27/5, 28/5, 29/5, 30/5, 31/5, 32/5, 24/5, 22/5, 20/5, 19/5, 18/5, 17/5, Inverter111/1, Inverter106/1, Inverter100/1, Inverter93/1, Inverter56/1, Inverter86/1, Inverter133/1
  Result41/1 -> Display72/1
  Inverter112/1 -> 9/2
  14/1 -> Convert42/1, Result38/1
  Result39/1 -> Display70/1
